simulink model "ball_and_plate"  (R2020a)
settings: Solver=ode23t  StartTime=0.0  StopTime=inf  RelTol=1e-3
model workspace (MAT data in the model file):
  L = 1
  d = 0.05
settings Model: PacingRate=0.110000  Creator=Mike  LastModifiedBy=janet

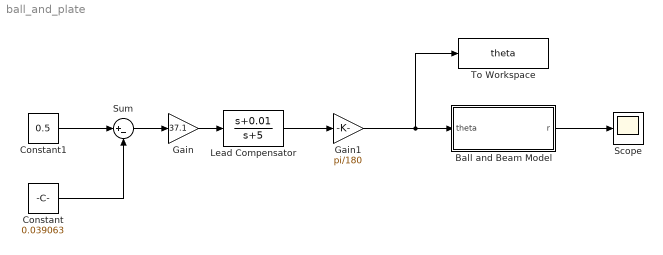
== system ball_and_plate ==
  Ball and Beam Model : Subsystem
  Constant : Constant  Value=0.039063
  Constant1 : Constant  Value=0.5
  Gain : Gain  Gain=37.1
      settings: AttributesFormatString=%<Gain>
  Gain1 : Gain  Gain=pi/180
      settings: AttributesFormatString=%<Gain>
  Lead Compensator : TransferFcn  Numerator=[1 0.01]  Denominator=[1 5]
      settings: AttributesFormatString=|
      | %<Numerator>
      | %<Denominator>
  Scope : Scope
  Sum : Sum  Inputs=|+-
  To Workspace : ToWorkspace  VariableName=theta  SaveFormat=Timeseries  SampleTime=-1
      settings: MaxDataPoints=1
  wires:
  Ball and Beam Model/1(r) -> Scope/1
  Lead Compensator/1 -> Gain1/1
  Gain/1 -> Lead Compensator/1
  Constant1/1 -> Sum/1
  Sum/1 -> Gain/1
  Constant/1 -> Sum/2
  Gain1/1 -> To Workspace/1, Ball and Beam Model/1(theta)

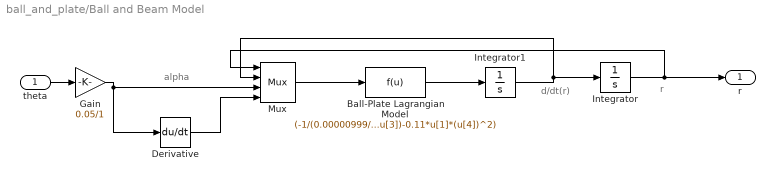
== system ball_and_plate/Ball and Beam Model ==
  note: alpha
  note: d/dt(r)
  note: r
  theta : Inport
  Ball-Plate Lagrangian Model : Fcn  Expr=(-1/(0.00000999/(0.5^2)+0.11))*(0.11*(-9.81)*sin(u[3])-0.11*u[1]*(u[4])^2)
  Derivative : Derivative
  Gain : Gain  Gain=0.05/1
  Integrator : Integrator
  Integrator1 : Integrator
  Mux : Mux
      settings: DisplayOption=signals
  r : Outport
  wires:
  Ball-Plate Lagrangian Model/1 -> Integrator1/1
  Mux/1 -> Ball-Plate Lagrangian Model/1
  Integrator1/1 -> Mux/2, Integrator/1
  theta/1 -> Gain/1
  Integrator/1 -> Mux/1, r/1
  Gain/1 -> Derivative/1, Mux/3
  Derivative/1 -> Mux/4
